simulink model "RollRW"  (R2017b)
settings: Solver=VariableStepAuto  StartTime=0.0  StopTime=10  RelTol=1e-3
undefined symbols (not defined in the file): Dphi, g, psi, radiusRW, sigbuilder_block, vec_n, X, xPla, Y, yPla, Z
libraries: nesl_utility x18, sm_lib x6, simulink x4, Contact_Forces_Lib x4, Parts_Lib x1
settings Model: Creator=r_ahmed_afzal  LastModifiedBy=r_ahmed_afzal

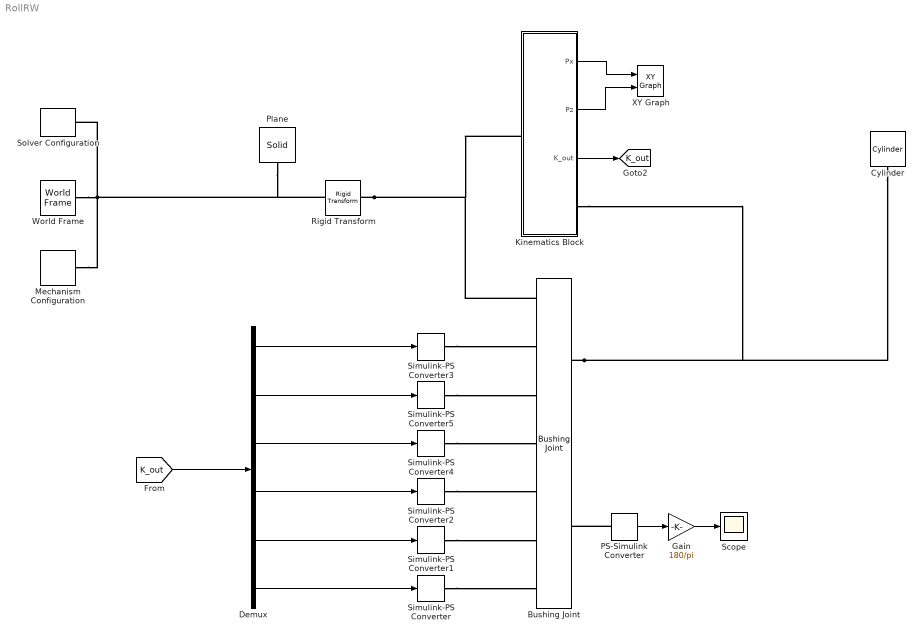
== system RollRW ==
  Bushing Joint : sm_lib/Joints/Bushing Joint  SenseConstraintForce=off  SenseConstraintForceX=off  SenseConstraintForceY=off  SenseConstraintForceZ=off  SenseConstraintTorque=off  SenseConstraintTorqueX=off  SenseConstraintTorqueY=off  SenseConstraintTorqueZ=off  SenseTotalForce=off  SenseTotalForceX=off  SenseTotalForceY=off  SenseTotalForceZ=off  SenseTotalTorque=off  SenseTotalTorqueX=off  SenseTotalTorqueY=off  SenseTotalTorqueZ=off  CompositeWrenchDir=FollowerOnBase  CompositeWrenchFrame=BaseFrame  PxEquilibriumPosition=0  PxEquilibriumPositionUnits=m  PxSpringStiffness=0  PxSpringStiffnessUnits=N/m  PxDampingCoefficient=0  PxDampingCoefficientUnits=N/(m/s)  PxTorqueActuationMode=ComputedTorque  PxMotionActuationMode=InputMotion  PxSensePosition=off  PxSenseVelocity=off  PxSenseAcceleration=off  PxSenseTorqueForce=off  PxPositionTargetSpecify=off  PxPositionTargetPriority=High  PxPositionTargetValue=0  PxPositionTargetValueUnits=m  PxVelocityTargetSpecify=off  PxVelocityTargetPriority=High  PxVelocityTargetValue=0  PxVelocityTargetValueUnits=m/s  PyEquilibriumPosition=-radiusRW  PyEquilibriumPositionUnits=m  PySpringStiffness=0  PySpringStiffnessUnits=N/m  PyDampingCoefficient=0  PyDampingCoefficientUnits=N/(m/s)  PyTorqueActuationMode=ComputedTorque  PyMotionActuationMode=InputMotion  PySensePosition=off  PySenseVelocity=off  PySenseAcceleration=off  PySenseTorqueForce=off  PyPositionTargetSpecify=on  PyPositionTargetPriority=High  PyPositionTargetValue=-radiusRW  PyPositionTargetValueUnits=m  PyVelocityTargetSpecify=off  PyVelocityTargetPriority=High  PyVelocityTargetValue=0  PyVelocityTargetValueUnits=m/s  PzEquilibriumPosition=0  PzEquilibriumPositionUnits=m  PzSpringStiffness=0  PzSpringStiffnessUnits=N/m  PzDampingCoefficient=0  PzDampingCoefficientUnits=N/(m/s)  PzTorqueActuationMode=ComputedTorque  PzMotionActuationMode=InputMotion  PzSensePosition=off  PzSenseVelocity=off  PzSenseAcceleration=off  PzSenseTorqueForce=off  PzPositionTargetSpecify=off  PzPositionTargetPriority=High  PzPositionTargetValue=0  PzPositionTargetValueUnits=m  PzVelocityTargetSpecify=off  PzVelocityTargetPriority=High  PzVelocityTargetValue=0  PzVelocityTargetValueUnits=m/s  RxEquilibriumPosition=0  RxEquilibriumPositionUnits=deg  RxSpringStiffness=0  RxSpringStiffnessUnits=N*m/deg  RxDampingCoefficient=0  RxDampingCoefficientUnits=N*m/(deg/s)  RxTorqueActuationMode=ComputedTorque  RxMotionActuationMode=InputMotion  RxSensePosition=on  RxSenseVelocity=off  RxSenseAcceleration=off  RxSenseTorqueForce=off  RxPositionTargetSpecify=off  RxPositionTargetPriority=High  RxPositionTargetValue=-10  RxPositionTargetValueUnits=deg  RxVelocityTargetSpecify=off  RxVelocityTargetPriority=High  RxVelocityTargetValue=0  RxVelocityTargetValueUnits=deg/s  RyEquilibriumPosition=0  RyEquilibriumPositionUnits=deg  RySpringStiffness=0  RySpringStiffnessUnits=N*m/deg  RyDampingCoefficient=0  RyDampingCoefficientUnits=N*m/(deg/s)  RyTorqueActuationMode=ComputedTorque  RyMotionActuationMode=InputMotion  RySensePosition=off  RySenseVelocity=off  RySenseAcceleration=off  RySenseTorqueForce=off  RyPositionTargetSpecify=off  RyPositionTargetPriority=High  RyPositionTargetValue=0  RyPositionTargetValueUnits=deg  RyVelocityTargetSpecify=off  RyVelocityTargetPriority=High  RyVelocityTargetValue=0  RyVelocityTargetValueUnits=deg/s  RzEquilibriumPosition=0  RzEquilibriumPositionUnits=deg  RzSpringStiffness=0  RzSpringStiffnessUnits=N*m/deg  RzDampingCoefficient=0  RzDampingCoefficientUnits=N*m/(deg/s)  RzTorqueActuationMode=ComputedTorque  RzMotionActuationMode=InputMotion  RzSensePosition=off  RzSenseVelocity=off  RzSenseAcceleration=off  RzSenseTorqueForce=off  RzPositionTargetSpecify=off  RzPositionTargetPriority=High  RzPositionTargetValue=0  RzPositionTargetValueUnits=deg  RzVelocityTargetSpecify=off  RzVelocityTargetPriority=High  RzVelocityTargetValue=0  RzVelocityTargetValueUnits=deg/s
      settings: SourceProductName=Simscape Multibody
  Cylinder : Parts_Lib/Cylinder  Tag=CustomStyle  cyl_radius=radiusRW  cyl_length=lengthRW  cyl_density=rhoRW  cyl_color=blue  cyl_opacity=1  cyl_color_custom="[0.7920    0.9900    0.9900]"  mark_radius=[0.75 0.5]  mark_len_factor=1.01  mark_angle=60  mark_color=purple  mark_opacity=1
  Demux : Demux  Outputs=6
  Gain : Gain  Gain=180/pi
  Kinematics Block : Subsystem
  Mechanism Configuration : sm_lib/Utilities/Mechanism Configuration  UniformGravity=Constant  GravityVector=[0 0 -g]  GravityUnits=m/s^2  LinearizationDelta=0.001
  PS-Simulink Converter : nesl_utility/PS-Simulink Converter  PhysicalDomain=network_engine_domain  SubClassName=ps_output  LeftPortType=input  RightPortType=output  PseudoPeriodic=off  Frequencies=[]  Unit=1  AffineConversion=off
  Plane : sm_lib/Body Elements/Solid  InertiaType=CalculateFromGeometry  Mass=1  MassUnits=kg  CenterOfMass=[0 0 0]  CenterOfMassUnits=m  MomentsOfInertia=[1 1 1]  MomentsOfInertiaUnits=kg*m^2  ProductsOfInertia=[1 1 1]  ProductsOfInertiaUnits=kg*m^2  DensityBased=on  Density=1000  DensityUnits=kg/m^3  DoExposeReferenceFrame=on  SerializedFrames=<Frames/>  GraphicType=FromGeometry  MarkerShape=Sphere  MarkerSize=10  GraphicVisPropType=SimpleVisualProperties  GraphicDiffuseColor=[0.5 0.5 0.5]  GraphicSpecularColor=[0.5 0.5 0.5 1.0]  GraphicAmbientColor=[0.15 0.15 0.15 1.0]  GraphicEmissiveColor=[0.0 0.0 0.0 1.0]  GraphicShininess=75  GraphicOpacity=0.5  GeometryShape=Brick  RectangleSize=[1 1]  RectangleSizeUnits=m  BrickDimensions=[xPla yPla 0.01]  BrickDimensionUnits=m  CylinderRadius=1  CylinderRadiusUnits=m  CylinderLength=1  CylinderLengthUnits=m  SphereRadius=1  SphereRadiusUnits=m  EllipsoidRadii=[1 1 1]  EllipsoidRadiiUnits=m  ExtrusionCrossSection=[1 1; -1 1; -1 -1; 1 -1]  ExtrusionCrossSectionUnits=m  ExtrusionLength=1  ExtrusionLengthUnits=m  PolygonNumSides=3  PolygonOuterRadius=1  PolygonOuterRadiusUnits=m  ExtGeomFileType=STEP  ExtGeomFileUnits=m  RevolutionCrossSection=[1 1; 1 -1; 2 -1; 2 1]  RevolutionCrossSectionUnits=m  RevolutionExtent=Full  RevolutionAngle=180  RevolutionAngleUnits=deg
  Rigid Transform : sm_lib/Frames and Transforms/Rigid Transform  TranslationMethod=None  TranslationStandardOffset=0  TranslationLengthUnit=m  TranslationStandardAxis=+Z  TranslationCartesianOffset=[0 0 0]  TranslationROffset=0  TranslationROffsetUnits=m  TranslationZOffset=0  TranslationZOffsetUnits=m  TranslationThetaOffset=0  TranslationThetaOffsetUnits=deg  RotationMethod=AlignedAxes  RotationAngleUnits=deg  RotationStandardAxis=+Z  RotationAngle=0.0  RotationArbitraryAxis=[0 0 1]  FollAlignAxisA=+Z  BaseAlignAxisA=+Y  FollAlignAxisB=+X  BaseAlignAxisB=+X  RotationSequenceAxes=FollowerAxes  RotationSequence=XYX  RotationSequenceAngles=[0 0 0]  RotationSequenceAnglesUnits=deg  RotationMatrix=[1 0 0; 0 1 0; 0 0 1]
  Scope : Scope
  Simulink-PS Converter{,1..5} (6 alike) : nesl_utility/Simulink-PS Converter  PhysicalDomain=network_engine_domain  SubClassName=ps_input  LeftPortType=input  RightPortType=output  PseudoPeriodic=off  Frequencies=[]  NoiseDistribution=none  NoiseParameters=[]  Unit=1  AffineConversion=off  FilteringAndDerivatives=filter  SimscapeFilterOrder=2  InputFilterTimeConstant=0.001  UdotUserProvided=0
  Solver Configuration : nesl_utility/Solver Configuration  PhysicalDomain=network_engine_domain  SubClassName=solver  LeftPortType=input  RightPortType=generic  Accelerate=off  Tones=[]  Harmonics=[]  SimulateNoise=off  Profile=off  UseLocalSampling=off  EnableSwitchedLinearOptims=on  FrequencyDomain=off  UseCCode=off  RelTol=0.001  AbsTol=1e-06  MinStep=1e-09  ToWorkspace=off  RevertToSquareIcSolve=off  NumHomotopyIterations=100  PhasorMode=off  PhasorModeNumHarmonics=1  DoDC=off  ResidualTolerance=1e-09  UseLocalSolver=off  LocalSolverChoice=NE_BACKWARD_EULER_ADVANCER  LocalSolverSampleTime=0.001  DoFixedCost=off  MaxNonlinIter=3  MaxModeIter=2  LinearAlgebra=Sparse  DelaysMemoryBudget=1024  AutomaticFiltering=on  FilteringTimeConstant=0.001
  World Frame : sm_lib/Frames and Transforms/World Frame
  XY Graph : simulink/Sinks/XY Graph  xmin=0  xmax=8  ymin=0  ymax=8  st=-1
  tag scope: K_out=global
  wires:
  Kinematics Block/3(K_out) -> [K_out]
  Gain/1 -> Scope/1
  PS-Simulink Converter/1 -> Gain/1
  Demux/4 -> Simulink-PS Converter2/1
  Demux/5 -> Simulink-PS Converter1/1
  [K_out] -> Demux/1
  Demux/3 -> Simulink-PS Converter4/1
  Demux/1 -> Simulink-PS Converter3/1
  Demux/2 -> Simulink-PS Converter5/1
  Demux/6 -> Simulink-PS Converter/1
  Kinematics Block/1(Px) -> XY Graph/1
  Kinematics Block/2(Pz) -> XY Graph/2
  connections:
  Bushing Joint/RConn1 -- Cylinder/LConn1 -- Kinematics Block/RConn1
  Rigid Transform/RConn1 -- Bushing Joint/LConn1 -- Kinematics Block/LConn1
  World Frame/RConn1 -- Plane/RConn1 -- Rigid Transform/LConn1 -- Solver Configuration/RConn1 -- Mechanism Configuration/RConn1
  Simulink-PS Converter2/RConn1 -- Bushing Joint/LConn5
  Simulink-PS Converter1/RConn1 -- Bushing Joint/LConn6
  Simulink-PS Converter5/RConn1 -- Bushing Joint/LConn3
  PS-Simulink Converter/LConn1 -- Bushing Joint/RConn2
  Simulink-PS Converter3/RConn1 -- Bushing Joint/LConn2
  Simulink-PS Converter/RConn1 -- Bushing Joint/LConn7
  Simulink-PS Converter4/RConn1 -- Bushing Joint/LConn4

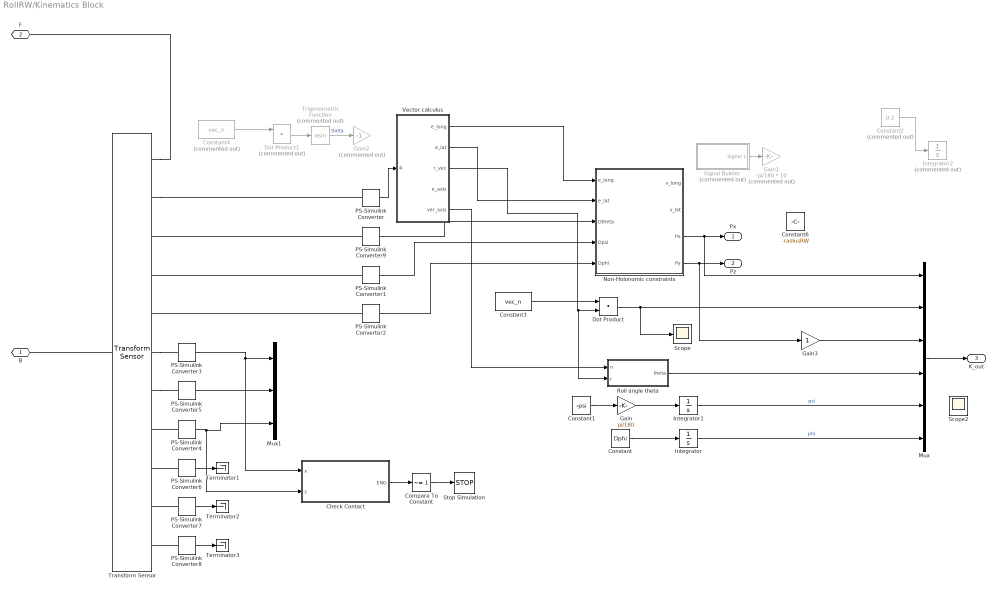
== system RollRW/Kinematics Block ==
  Check Contact : Subsystem
  Compare To Constant : simulink/Logic and Bit Operations/Compare To Constant  relop=~=  const=1  OutDataTypeStr=boolean
  Constant : Constant  Value=Dphi
  Constant1 : Constant  Value=-psi
  Constant2 : Constant  Commented=on  Value=0.1
  Constant3 : Constant  Value=vec_n
  Constant4 : Constant  Commented=on  Value=vec_n
  Constant6 : Constant  Value=-radiusRW
  Dot Product : DotProduct  InputSameDT=on  OutDataTypeStr=Inherit: Inherit via internal rule
  Dot Product1 : DotProduct  Commented=on  InputSameDT=on  OutDataTypeStr=Inherit: Inherit via internal rule
  Gain : Gain  Gain=pi/180
  Gain1 : Gain  Commented=on  Gain=-pi/180 * 10
  Gain2 : Gain  Commented=on  Gain=-1
  Gain3 : Gain
  Integrator : Integrator
  Integrator1 : Integrator
  Integrator2 : Integrator  Commented=on
  Mux : Mux  Inputs=6
  Mux1 : Mux  Inputs=3
  Non-Holonomic constraints : Subsystem
  PS-Simulink Converter{,1..9} (10 alike) : nesl_utility/PS-Simulink Converter  PhysicalDomain=network_engine_domain  SubClassName=ps_output  LeftPortType=input  RightPortType=output  PseudoPeriodic=off  Frequencies=[]  Unit=1  AffineConversion=off
  Roll angle theta : Subsystem
  Scope : Scope
  Scope2 : Scope
  Signal Builder : Subsystem  Tag=STV Subsys  Commented=on  LoadFcn=sigbuilder_block('load');  StartFcn=sigbuilder_block('start');  StopFcn=sigbuilder_block('stop');  ClipboardFcn=sigbuilder_block('clipboard');  mask(Sigbuilder block){tuvar=[0:10]}
      mask help: Simulink:masks:SigbuilderBlock_MD
      mask init:
      | if ~strcmp(get_param(bdroot(gcbh),'SimulationStatus'),'stopped') tuvar = sigbuilder_block('maskInit'); end
      settings: CopyFcn=sigbuilder_block('copy');  DeleteFcn=sigbuilder_block('delete');  ModelCloseFcn=sigbuilder_block('modelClose');  PreSaveFcn=sigbuilder_block('preSave');  PauseFcn=sigbuilder_block('pause');  ContinueFcn=sigbuilder_block('continue');  NameChangeFcn=sigbuilder_block('namechange');  OpenFcn=sigbuilder_block('open',[437.6 199.2 550.4 400 ]);  CloseFcn=sigbuilder_block('close');
      mask Display: plot(0, 0, 100, 100,[2, 2, 32, 32, 2], [68, 8, 8, 68, 68],[32, 2], [38, 38], [32, 19, 2],[53, 60, 44], [32, 17, 17, 2],[16, 16, 31, 31]);txt = getActiveGroup(gcbh);text(2, 100, txt,'verticalAlignment', 'top');
  Stop Simulation : Stop
  Terminator1 : Terminator
  Terminator2 : Terminator
  Terminator3 : Terminator
  Transform Sensor : sm_lib/Frames and Transforms/Transform Sensor  MeasurementFrame=Follower  SenseAngle=off  SenseAxis=off  SenseAngle1=off  SenseAngle2=off  SenseAngle3=off  SenseQ=off  SenseR=on  SenseOmegaX=on  SenseOmegaY=on  SenseOmegaZ=on  SenseOmega1=off  SenseOmega2=off  SenseOmega3=off  SenseQDot=off  SenseRDot=off  SenseAlphaX=off  SenseAlphaY=off  SenseAlphaZ=off  SenseAlpha1=off  SenseAlpha2=off  SenseAlpha3=off  SenseQDDot=off  SenseRDDot=off  SenseX=on  SenseY=on  SenseZ=on  SenseRad=off  SenseAzim=off  SenseDist=off  SenseInc=off  SenseXDot=on  SenseYDot=on  SenseZDot=on  SenseRadDot=off  SenseAzimDot=off  SenseDistDot=off  SenseIncDot=off  SenseXDDot=off  SenseYDDot=off  SenseZDDot=off  SenseRadDDot=off  SenseAzimDDot=off  SenseDistDDot=off  SenseIncDDot=off
  Trigonometric Function : Trigonometry  Commented=on  Operator=asin
  Vector calculus : Subsystem
  B : PMIOPort  Port=1  Side=Left
  F : PMIOPort  Port=2  Side=Right
  Px : Outport
  Pz : Outport  Port=2
  K_out : Outport  Port=3
  wires:
  PS-Simulink Converter3/1 -> Mux1/1, Check Contact/1(x)
  PS-Simulink Converter4/1 -> Mux1/3, Check Contact/2(z)
  Vector calculus/1(e_long) -> Non-Holonomic constraints/1(e_long)
  Vector calculus/2(e_lat) -> Non-Holonomic constraints/2(e_lat)
  PS-Simulink Converter/1 -> Vector calculus/1(R)
  Integrator/1 -> Mux/6  "phi"
  Trigonometric Function/1 -> Gain2/1  "theta"
  Mux/1 -> K_out/1
  Check Contact/1(ENG) -> Compare To Constant/1
  Compare To Constant/1 -> Stop Simulation/1
  PS-Simulink Converter2/1 -> Non-Holonomic constraints/5(Dphi)
  Dot Product1/1 -> Trigonometric Function/1
  PS-Simulink Converter5/1 -> Mux1/2
  PS-Simulink Converter6/1 -> Terminator1/1
  PS-Simulink Converter7/1 -> Terminator2/1
  PS-Simulink Converter8/1 -> Terminator3/1
  Signal Builder/1(Signal 1) -> Gain1/1
  Constant4/1 -> Dot Product1/1
  Vector calculus/3(r_vec) -> Roll angle theta/2(r), Dot Product/2
  Constant2/1 -> Integrator2/1
  Dot Product/1 -> Mux/2, Scope/1
  Non-Holonomic constraints/3(Px) -> Mux/1, Px/1
  Non-Holonomic constraints/4(Py) -> Gain3/1, Pz/1
  PS-Simulink Converter9/1 -> Non-Holonomic constraints/3(Dtheta)
  PS-Simulink Converter1/1 -> Non-Holonomic constraints/4(Dpsi)
  Constant1/1 -> Gain/1
  Roll angle theta/1(theta) -> Mux/4
  Constant3/1 -> Dot Product/1
  Integrator1/1 -> Mux/5  "psi"
  Gain3/1 -> Mux/3
  Constant/1 -> Integrator/1
  Gain/1 -> Integrator1/1
  Vector calculus/5(ver_axis) -> Roll angle theta/1(n)
  connections:
  Transform Sensor/LConn1 -- B/RConn1
  Transform Sensor/RConn1 -- F/RConn1
  Transform Sensor/RConn2 -- PS-Simulink Converter/LConn1
  PS-Simulink Converter2/LConn1 -- Transform Sensor/RConn5
  PS-Simulink Converter1/LConn1 -- Transform Sensor/RConn4
  Transform Sensor/RConn6 -- PS-Simulink Converter3/LConn1
  PS-Simulink Converter4/LConn1 -- Transform Sensor/RConn8
  Transform Sensor/RConn7 -- PS-Simulink Converter5/LConn1
  PS-Simulink Converter6/LConn1 -- Transform Sensor/RConn9
  PS-Simulink Converter7/LConn1 -- Transform Sensor/RConn10
  PS-Simulink Converter8/LConn1 -- Transform Sensor/RConn11
  PS-Simulink Converter9/LConn1 -- Transform Sensor/RConn3

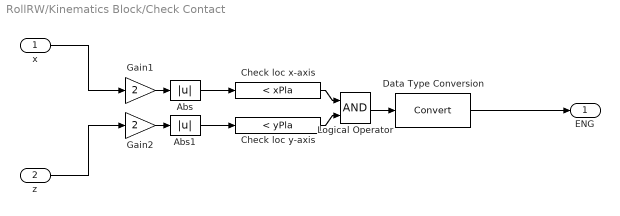
== system RollRW/Kinematics Block/Check Contact ==
  x : Inport
  z : Inport  Port=2
  Abs : Abs  ZeroCross=off
  Abs1 : Abs  ZeroCross=off
  Check loc x-axis : simulink/Logic and Bit Operations/Compare To Constant  relop=<  const=xPla  OutDataTypeStr=boolean  ZeroCross=off
  Check loc y-axis : simulink/Logic and Bit Operations/Compare To Constant  relop=<  const=yPla  OutDataTypeStr=boolean  ZeroCross=off
  Data Type Conversion : DataTypeConversion
  Gain1 : Gain  Gain=2
  Gain2 : Gain  Gain=2
  Logical Operator : Logic  AllPortsSameDT=off  OutDataTypeStr=boolean
  ENG : Outport
  wires:
  x/1 -> Gain1/1
  Gain1/1 -> Abs/1
  Check loc x-axis/1 -> Logical Operator/1
  Abs1/1 -> Check loc y-axis/1
  Gain2/1 -> Abs1/1
  Logical Operator/1 -> Data Type Conversion/1
  z/1 -> Gain2/1
  Data Type Conversion/1 -> ENG/1
  Check loc y-axis/1 -> Logical Operator/2
  Abs/1 -> Check loc x-axis/1

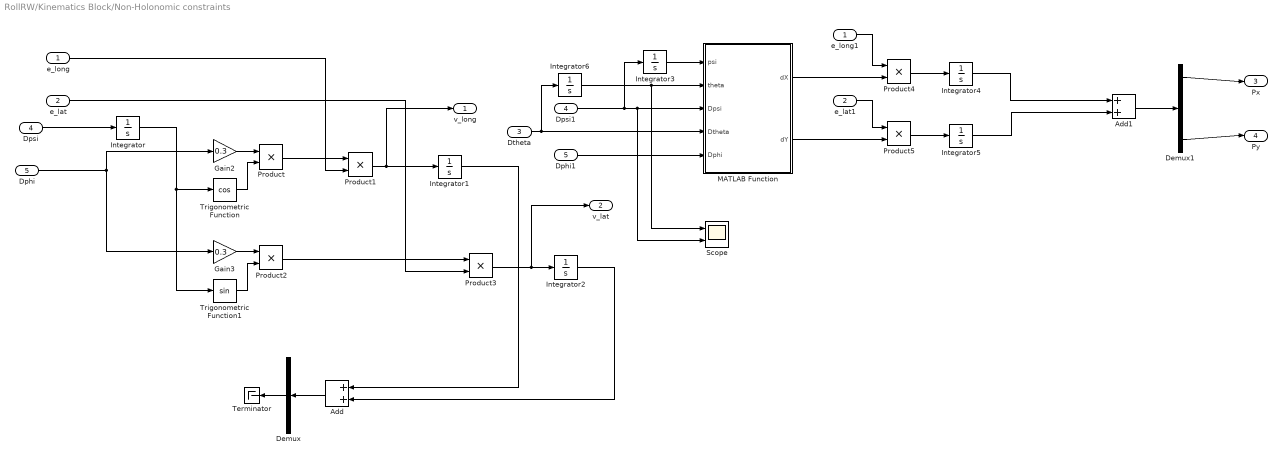
== system RollRW/Kinematics Block/Non-Holonomic constraints ==
  e_long : Inport
  e_lat : Inport  Port=2
  Dtheta : Inport  Port=3
  Dpsi : Inport  Port=4
  Dphi : Inport  Port=5
  Add : Sum  Inputs=2
  Add1 : Sum
  Demux : Demux  Outputs=3
  Demux1 : Demux  Outputs=3
  Dphi1 : InportShadow  Port=5
  Dpsi1 : InportShadow  Port=4
  Gain2 : Gain  Gain=0.3
  Gain3 : Gain  Gain=0.3
  Integrator{,1..6} (7 alike) : Integrator
  MATLAB Function : MATLAB Function  TreatAsAtomicUnit=on
  Product{,1..5} (6 alike) : Product
  Scope : Scope  NumInputPorts=2
  Terminator : Terminator
  Trigonometric Function : Trigonometry  Operator=cos
  Trigonometric Function1 : Trigonometry
  e_lat1 : InportShadow  Port=2
  e_long1 : InportShadow
  v_long : Outport
  v_lat : Outport  Port=2
  Px : Outport  Port=3
  Py : Outport  Port=4
  wires:
  Dphi/1 -> Gain2/1, Gain3/1
  Dpsi/1 -> Integrator/1
  Integrator1/1 -> Add/1
  Demux/2 -> Terminator/1
  e_long/1 -> Product1/2
  Add/1 -> Demux/1
  Integrator2/1 -> Add/2
  e_lat/1 -> Product3/2
  Product/1 -> Product1/1
  Gain2/1 -> Product/1
  Trigonometric Function/1 -> Product/2
  Trigonometric Function1/1 -> Product2/2
  Gain3/1 -> Product2/1
  Integrator/1 -> Trigonometric Function1/1, Trigonometric Function/1
  Product1/1 -> v_long/1, Integrator1/1
  Product2/1 -> Product3/1
  Product3/1 -> v_lat/1, Integrator2/1
  Dpsi1/1 -> Integrator3/1, Scope/2, MATLAB Function/3(Dpsi)
  Dphi1/1 -> MATLAB Function/5(Dphi)
  Integrator3/1 -> MATLAB Function/1(psi)
  Integrator6/1 -> Scope/1, MATLAB Function/2(theta)
  Dtheta/1 -> Integrator6/1, MATLAB Function/4(Dtheta)
  MATLAB Function/1(dX) -> Product4/2
  e_long1/1 -> Product4/1
  MATLAB Function/2(dY) -> Product5/2
  e_lat1/1 -> Product5/1
  Product4/1 -> Integrator4/1
  Product5/1 -> Integrator5/1
  Add1/1 -> Demux1/1
  Demux1/1 -> Px/1
  Demux1/3 -> Py/1
  Integrator4/1 -> Add1/1
  Integrator5/1 -> Add1/2

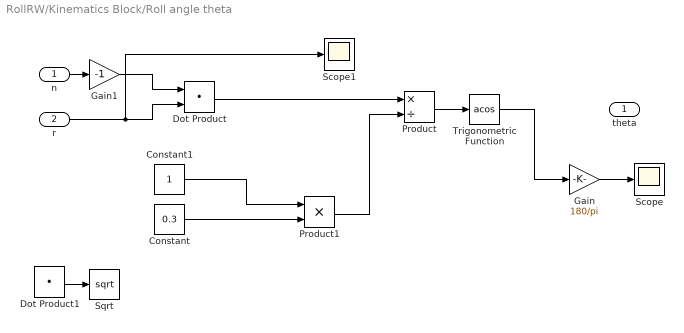
== system RollRW/Kinematics Block/Roll angle theta ==
  n : Inport
  r : Inport  Port=2
  Constant : Constant  Value=0.3
  Constant1 : Constant
  Dot Product : DotProduct  InputSameDT=on  OutDataTypeStr=Inherit: Inherit via internal rule
  Dot Product1 : DotProduct  InputSameDT=on  OutDataTypeStr=Inherit: Inherit via internal rule
  Gain : Gain  Gain=180/pi
  Gain1 : Gain  Gain=-1
  Product : Product  Inputs=*/
  Product1 : Product
  Scope : Scope
  Scope1 : Scope
  Sqrt : Sqrt  SaturateOnIntegerOverflow=on
  Trigonometric Function : Trigonometry  Operator=acos
  theta : Outport
  wires:
  n/1 -> Gain1/1
  Dot Product/1 -> Product/1
  Dot Product1/1 -> Sqrt/1
  Product1/1 -> Product/2
  Product/1 -> Trigonometric Function/1
  r/1 -> Scope1/1, Dot Product/2
  Gain/1 -> Scope/1
  Trigonometric Function/1 -> Gain/1
  Gain1/1 -> Dot Product/1
  Constant1/1 -> Product1/1
  Constant/1 -> Product1/2

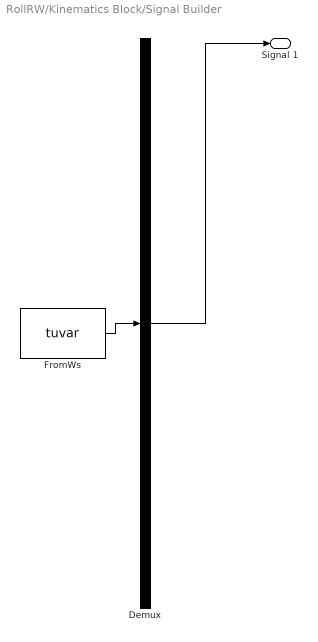
== system RollRW/Kinematics Block/Signal Builder ==
  Demux : Demux  Tag=STV Demux  Outputs=1
  FromWs : FromWorkspace  Tag=STV FromWs  VariableName=tuvar  SampleTime=0
      SigBuilderData=|
      | common.afterFinalStr = 'Extrapolate'
      | common.sampleTime = 0
      | dataSet.timeRange = [0 10]
      | dataSet.name = 'Group 1'
      | sbobj.Groups.Name = 'Group 1'
      | sbobj.Groups.Signals.Name = 'Signal 1'
      | sbobj.Groups.Signals.XData = [0 0.5 0.5 10]
      | sbobj.Groups.Signals.YData = [1 1 0 0]
  Signal 1 : Outport  Tag=STV Outport
  wires:
  Demux/1 -> Signal 1/1
  FromWs/1 -> Demux/1

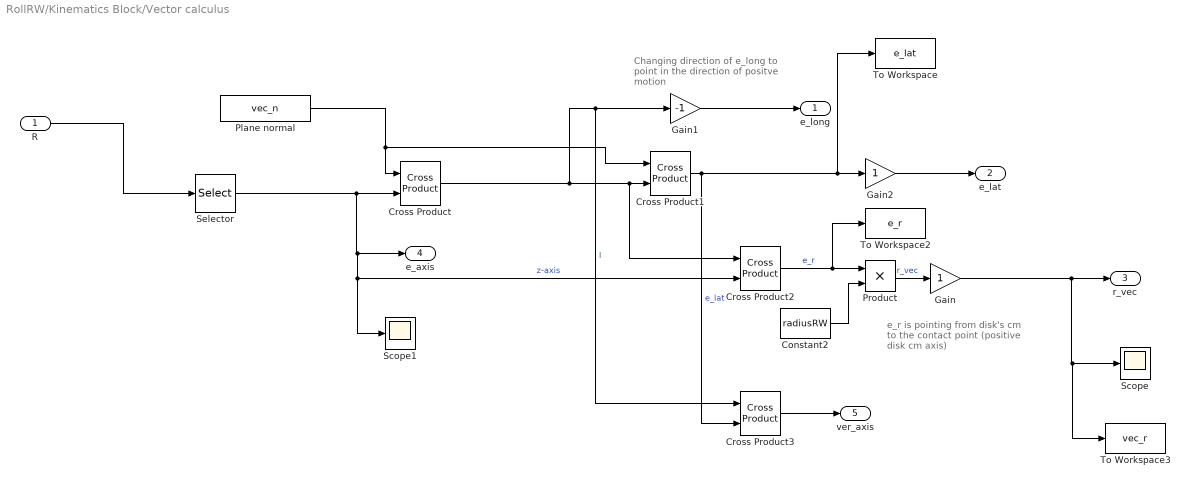
== system RollRW/Kinematics Block/Vector calculus ==
  note: Changing direction of e_long
      | to point in the direction of positve
      | motion
  note: e_r is pointing from
      | disk's cm to the
      | contact point
      |
      | (positive disk cm axis)
  R : Inport
  Constant2 : Constant  Value=radiusRW
  Cross Product{,1..3} (4 alike) : Contact_Forces_Lib/Math/Cross Product
  Gain : Gain
  Gain1 : Gain  Gain=-1
  Gain2 : Gain
  Plane normal : Constant  Value=vec_n
  Product : Product
  Scope : Scope
  Scope1 : Scope
  Selector : Selector  NumberOfDimensions=2  InputPortWidth=3  IndexOptions=Select all,Index vector (dialog)  Indices=[1 3],3  OutputSizes=1,1
  To Workspace : ToWorkspace  VariableName=e_lat  SaveFormat=Timeseries  SampleTime=-1
  To Workspace2 : ToWorkspace  VariableName=e_r  SaveFormat=Timeseries  SampleTime=-1
  To Workspace3 : ToWorkspace  VariableName=vec_r  SaveFormat=Timeseries  SampleTime=-1
  e_long : Outport
  e_lat : Outport  Port=2
  r_vec : Outport  Port=3
  e_axis : Outport  Port=4
  ver_axis : Outport  Port=5
  wires:
  Constant2/1 -> Product/2
  Product/1 -> Gain/1  "r_vec"
  Cross Product2/1 -> To Workspace2/1, Product/1  "e_r"
  Cross Product1/1 -> Cross Product3/2, To Workspace/1, Gain2/1  "e_lat"
  Selector/1 -> Scope1/1, Cross Product2/2, e_axis/1, Cross Product/2  "z-axis"
  Cross Product/1 -> Cross Product3/1, Gain1/1, Cross Product2/1, Cross Product1/2  "l"
  R/1 -> Selector/1
  Plane normal/1 -> Cross Product/1, Cross Product1/1
  Gain1/1 -> e_long/1
  Gain2/1 -> e_lat/1
  Gain/1 -> To Workspace3/1, Scope/1, r_vec/1
  Cross Product3/1 -> ver_axis/1

== matlab function RollRW/Kinematics Block/Non-Holonomic constraints/MATLAB Function ==
  data: dX output; psi input; theta input; Dpsi input; Dtheta input; Dphi input; dY output; radiusRW parameter
function [dX,dY] = fcn(psi, theta, Dpsi, Dtheta,Dphi,radiusRW)
R = radiusRW;
dX = (R * cos(psi))*Dphi - (R * sin(theta) * cos(psi) * Dpsi) - (R * cos(theta) * sin(psi) * Dtheta);
dY = (R * sin(psi))*Dphi - (R * sin(theta) * sin(psi) * Dpsi) + (R * cos(theta) * cos(psi) * Dtheta);

%dX = (R * cos(psi))*Dphi;
%dY = (R * sin(psi))*Dphi;
end
